simulink subsystem "ModeleNonLineaire"  (R2023a)
settings: Solver=VariableStepAuto  StartTime=0.0  StopTime=10.0  RelTol=1e-3
settings Model: Creator=raphb  LastModifiedBy=raphb

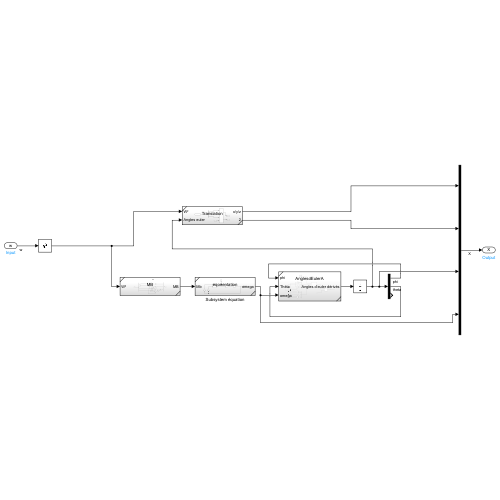
[thumbnail: Simulink's stored preview of the top-level diagram]
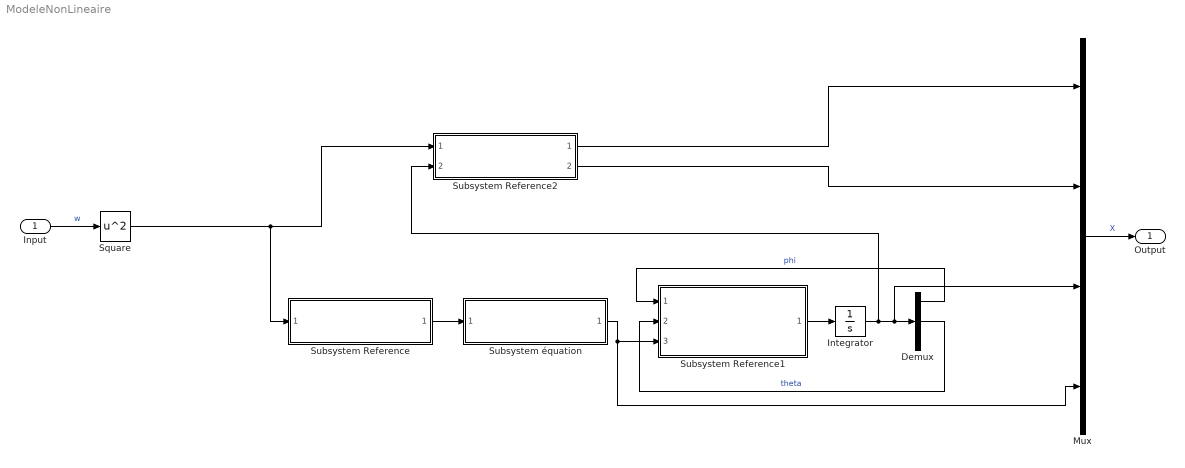
== system ModeleNonLineaire ==
  Input : Inport  PortDimensions=4
  Demux : Demux  Outputs=3
  Integrator : Integrator
  Mux : Mux
  Square : Math  Operator=square
  Subsystem Reference : Subsystem  ReferencedSubsystem=MB
  Subsystem Reference1 : Subsystem  ReferencedSubsystem=AnglesdEulerA
  Subsystem Reference2 : Subsystem  ReferencedSubsystem=Translation
  Subsystem équation : Subsystem  ReferencedSubsystem=eqorientation
  Output : Outport
  wires:
  Demux/1 -> Subsystem Reference1/1  "phi"
  Square/1 -> Subsystem Reference/1, Subsystem Reference2/1
  Subsystem Reference/1 -> Subsystem équation/1
  Subsystem Reference1/1 -> Integrator/1
  Demux/2 -> Subsystem Reference1/2  "theta"
  Integrator/1 -> Subsystem Reference2/2, Mux/3, Demux/1
  Input/1 -> Square/1  "w"
  Mux/1 -> Output/1  "X"
  Subsystem Reference2/1 -> Mux/1
  Subsystem Reference2/2 -> Mux/2
  Subsystem équation/1 -> Mux/4, Subsystem Reference1/3
